simulink model "float_sch_SWTTEO"  (R2020a)
settings: Solver=VariableStepAuto  StartTime=0  StopTime=5  RelTol=1e-3
values from neighbouring files (symbols this model uses):
  buffer_hamming_length = hamming_w_length    (= 32)    [float_sch_run_SWTTEO.m]
  feature_buffer = fs    (= 30000)    [float_sch_run_SNEO.m]    (also in float_sch_run_SWTTEO.m)
  feature_gain = [1]    [float_sch_run_SNEO.m]    (also in float_sch_run_SWTTEO.m = [3])
  fs = 30000    [float_sch_run_SNEO.m]    (also in float_sch_run_SWTTEO.m)
  hamming_w_length = 32    [float_sch_run_SWTTEO.m]
  refractory = 10^-3    (= 0.001)    [float_sch_run_SNEO.m]    (also in float_sch_run_SWTTEO.m)
  TEO_buffer = w_smooth    (= 30)    [float_sch_run_SNEO.m]    (also in float_sch_run_SWTTEO.m = length(wav_approx)-1)
libraries: dsparch4 x2, dspsigops x2, dspswit3 x1, dspstat3 x1, simulink x1, hdlsllib x1
settings Model: PauseTimes=2  Creator=diflo  LastModifiedBy=diflo

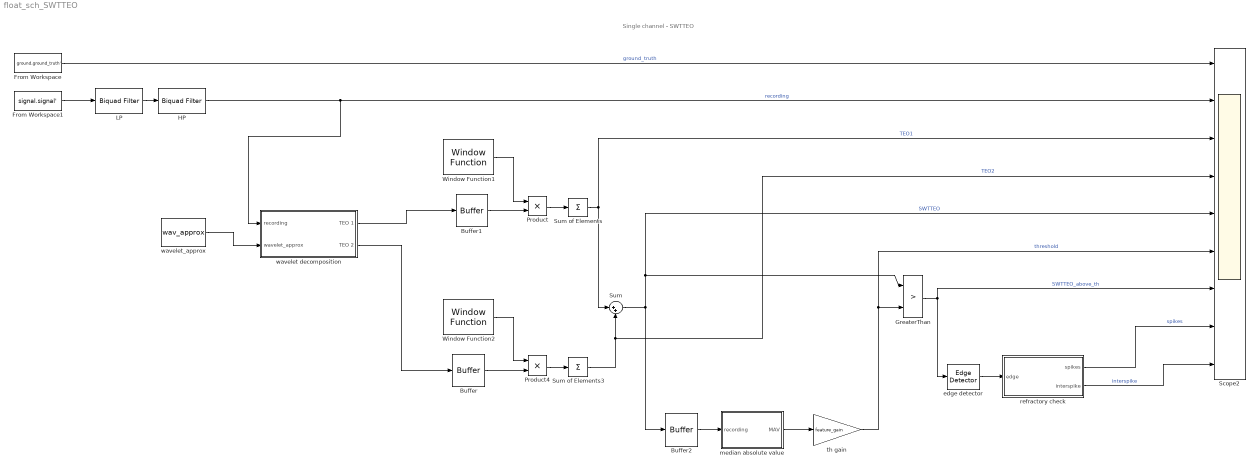
== system float_sch_SWTTEO ==
  note: Single channel - SWTTEO
  Buffer : Buffer  N=buffer_hamming_length  V=buffer_hamming_length_overlap  OutputFrames=off
  Buffer1 : Buffer  N=buffer_hamming_length  V=buffer_hamming_length_overlap  OutputFrames=off
  Buffer2 : Buffer  N=feature_buffer  OutputFrames=off
  From Workspace : FromWorkspace  VariableName=ground.ground_truth'  SampleTime=1/fs
  From Workspace1 : FromWorkspace  VariableName=signal.signal'  SampleTime=1/fs
  GreaterThan : RelationalOperator  Operator=>  OutDataTypeStr=boolean  RndMeth=Simplest
  HP : dsparch4/Biquad Filter  Tag=BlockMethodSubSystem  FilterSource=Dialog parameters  CoeffSource=Specify via dialog  FilterObject=BQF  IIRFiltStruct=Direct form II  BiQuadCoeffs=[1 -2 1 1 -1.93529438685999167 0.93912079880642374;1 -1 0 1 -0.939062505817492399 0]  ScaleValues=[0.968603796416603768;0.969531252908746199;1]  IC=0  ICnum=0  ICden=0  a0Flag=Warning  optimizeScaleValues=on  ScaleValueMode=Specify via input port (g)  roundingMode=Floor  overflowMode=off  scaleValueFracLength=14  denProdOutputFracLength=30  denAccumFracLength=30  secondMemoryFracLength=15
  LP : dsparch4/Biquad Filter  Tag=BlockMethodSubSystem  FilterSource=Dialog parameters  CoeffSource=Specify via dialog  FilterObject=BQF  IIRFiltStruct=Direct form II  BiQuadCoeffs=[1 1 0 1 -0.509525449494428795 0]  ScaleValues=[0.245237275252785547;1]  IC=0  ICnum=0  ICden=0  a0Flag=Warning  optimizeScaleValues=on  ScaleValueMode=Specify via input port (g)  roundingMode=Floor  overflowMode=off  scaleValueFracLength=14  denProdOutputFracLength=30  denAccumFracLength=30  secondMemoryFracLength=15
  Product : Product
  Product4 : Product
  Scope2 : Scope  NumInputPorts=9
  Sum : Sum  Inputs=|++
  Sum of Elements : Sum  Inputs=+
  Sum of Elements3 : Sum  Inputs=+
  Window Function1 : dspsigops/Window Function  winmode=Generate window  wintype=Hamming  sampmode=Discrete  samptime=1/fs  N=hamming_w_length  Rs=50  beta=10  winsamp=Symmetric  UserWindow=hamming  OptParams=off  UserParams={'symmetric'}  dataType=double  isSigned=on  wordLen=16  udDataType=sfix(16)  fracBitsMode=Best precision  numFracBits=15  roundingMode=Floor  overflowMode=off  numSidelobes=4  sidelobeLevel=-30
      settings: SourceProductBaseCode=DS
  Window Function2 : dspsigops/Window Function  winmode=Generate window  wintype=Hamming  sampmode=Discrete  samptime=1/fs  N=hamming_w_length  Rs=50  beta=10  winsamp=Symmetric  UserWindow=hamming  OptParams=off  UserParams={'symmetric'}  dataType=double  isSigned=on  wordLen=16  udDataType=sfix(16)  fracBitsMode=Best precision  numFracBits=15  roundingMode=Floor  overflowMode=off  numSidelobes=4  sidelobeLevel=-30
      settings: SourceProductBaseCode=DS
  edge detector : dspswit3/Edge Detector  InputProcessing=Columns as channels (frame based)
      settings: SourceProductBaseCode=DS
  median absolute value : Subsystem
  refractory check : Subsystem
  th gain : Gain  Gain=feature_gain
  wavelet decomposition : Subsystem
  wavelet_approx : FromWorkspace  VariableName=wav_approx  SampleTime=1/fs
  wires:
  Product/1 -> Sum of Elements/1
  wavelet decomposition/1(TEO 1) -> Buffer1/1
  Window Function1/1 -> Product/1
  Window Function2/1 -> Product4/1
  wavelet decomposition/2(TEO 2) -> Buffer/1
  Product4/1 -> Sum of Elements3/1
  Sum of Elements/1 -> Scope2/3, Sum/1  "TEO1"
  Sum of Elements3/1 -> Sum/2, Scope2/4  "TEO2"
  wavelet_approx/1 -> wavelet decomposition/2(wavelet_approx)
  Sum/1 -> Scope2/5, GreaterThan/1, Buffer2/1  "SWTTEO"
  median absolute value/1(MAV) -> th gain/1
  th gain/1 -> Scope2/6, GreaterThan/2  "threshold"
  GreaterThan/1 -> edge detector/1, Scope2/7  "SWTTEO_above_th"
  edge detector/1 -> refractory check/1("  edge ")
  refractory check/1(spikes) -> Scope2/8  "spikes"
  refractory check/2(interspike) -> Scope2/9  "interspike"
  Buffer/1 -> Product4/2
  Buffer1/1 -> Product/2
  Buffer2/1 -> median absolute value/1(recording)
  HP/1 -> wavelet decomposition/1(recording), Scope2/2  "recording"
  From Workspace1/1 -> LP/1
  From Workspace/1 -> Scope2/1  "ground_truth"
  LP/1 -> HP/1

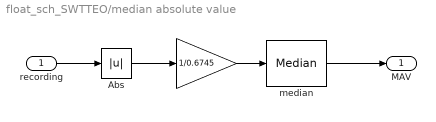
== system float_sch_SWTTEO/median absolute value ==
  recording : Inport
  "  " : Gain  Gain=1/0.6745
  Abs : Abs
  median : dspstat3/Median  sortAlg=Quick sort  directionMode=Each column  dimension=1  roundingMode=Floor  overflowMode=off  accumDataTypeStr=Inherit: Same as product output  accumLastDataTypeStr=Inherit: Same as product output  outputDataTypeStr=Inherit: Same as accumulator  outputMin=[]  outputMax=[]  outputLastDataTypeStr=Inherit: Same as accumulator
      settings: SourceProductBaseCode=DS  allowOverrides=off
  MAV : Outport
  wires:
  Abs/1 -> "  "/1
  "  "/1 -> median/1
  recording/1 -> Abs/1
  median/1 -> MAV/1

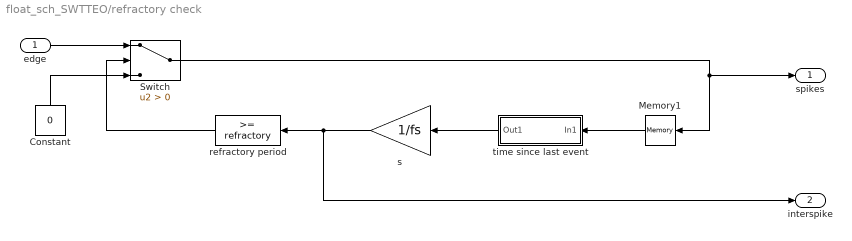
== system float_sch_SWTTEO/refractory check ==
  "  edge " : Inport
  Constant : Constant  Value=0
  Memory1 : Memory  InheritSampleTime=on
  Switch : Switch  Criteria=u2 > Threshold
  refractory period : simulink/Logic and Bit Operations/Compare To Constant  relop=>=  const=refractory  OutDataTypeStr=boolean
  s : Gain  Gain=1/fs  ParamDataTypeStr=double
  time since last event : Subsystem
  spikes : Outport
  interspike : Outport  Port=2
  wires:
  "  edge "/1 -> Switch/1
  Memory1/1 -> time since last event/1(In1)
  time since last event/1(Out1) -> s/1
  Constant/1 -> Switch/3
  s/1 -> refractory period/1, interspike/1
  Switch/1 -> spikes/1, Memory1/1
  refractory period/1 -> Switch/2

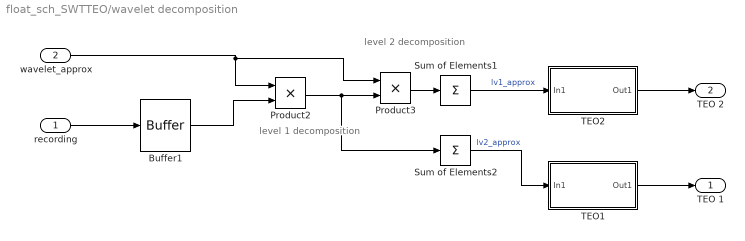
== system float_sch_SWTTEO/wavelet decomposition ==
  note: level 1
      | decomposition
  note: level 2
      | decomposition
  recording : Inport
  wavelet_approx : Inport  Port=2
  Buffer1 : Buffer  N=TEO_buffer  V=TEO_buffer_overlap  OutputFrames=off
  Product2 : Product
  Product3 : Product
  Sum of Elements1 : Sum  Inputs=+
  Sum of Elements2 : Sum  Inputs=+
  TEO1 : Subsystem
  TEO2 : Subsystem
  TEO 1 : Outport
  TEO 2 : Outport  Port=2
  wires:
  Sum of Elements1/1 -> TEO2/1(In1)  "lv1_approx"
  wavelet_approx/1 -> Product2/1, Product3/1
  Product3/1 -> Sum of Elements1/1
  Product2/1 -> Product3/2, Sum of Elements2/1
  TEO1/1(Out1) -> TEO 1/1
  TEO2/1(Out1) -> TEO 2/1
  Sum of Elements2/1 -> TEO1/1(In1)  "lv2_approx"
  Buffer1/1 -> Product2/2
  recording/1 -> Buffer1/1

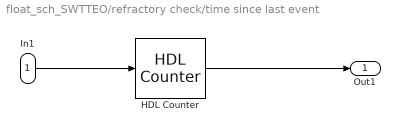
== system float_sch_SWTTEO/refractory check/time since last event ==
  In1 : Inport
  HDL Counter : hdlsllib/Sources/HDL Counter  CountType=Free running  CountInit=1  CountStep=1  CountMax=25  CountFromType=Initial value  CountFrom=1  CountResetPort=on  CountLoadPort=off  CountEnbPort=off  CountDirPort=off  CountDataType=Unsigned  CountWordLen=32  CountFracLen=0  CountSampTime=1
  Out1 : Outport
  wires:
  In1/1 -> HDL Counter/1
  HDL Counter/1 -> Out1/1

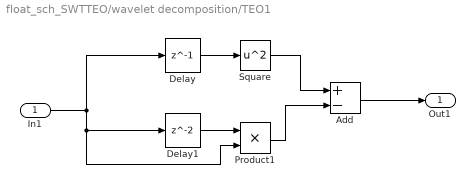
== system float_sch_SWTTEO/wavelet decomposition/TEO1 ==
  In1 : Inport
  Add : Sum  Inputs=+-
  Delay : Delay  DelayLength=1  InitialCondition=0  SampleTime=1/30000
  Delay1 : Delay  InitialCondition=0  SampleTime=1/30000
  Product1 : Product
  Square : Math  Operator=square  SaturateOnIntegerOverflow=on
  Out1 : Outport
  wires:
  Delay1/1 -> Product1/1
  Square/1 -> Add/1
  Add/1 -> Out1/1
  Delay/1 -> Square/1
  Product1/1 -> Add/2
  In1/1 -> Delay/1, Delay1/1, Product1/2

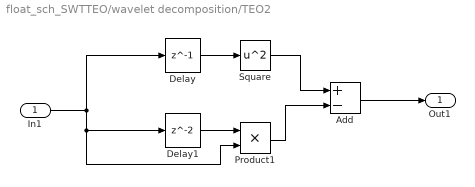
== system float_sch_SWTTEO/wavelet decomposition/TEO2 ==
  In1 : Inport
  Add : Sum  Inputs=+-
  Delay : Delay  DelayLength=1  InitialCondition=0  SampleTime=1/30000
  Delay1 : Delay  InitialCondition=0  SampleTime=1/30000
  Product1 : Product
  Square : Math  Operator=square  SaturateOnIntegerOverflow=on
  Out1 : Outport
  wires:
  Delay1/1 -> Product1/1
  Square/1 -> Add/1
  Add/1 -> Out1/1
  Delay/1 -> Square/1
  Product1/1 -> Add/2
  In1/1 -> Delay/1, Delay1/1, Product1/2
